simulink model "sys2"  (R2023b)
settings: Solver=VariableStepAuto  StartTime=0.0  StopTime=10.0  RelTol=1e-3
undefined symbols (not defined in the file): sys2
settings Model: Creator=lopez  LastModifiedBy=lopez

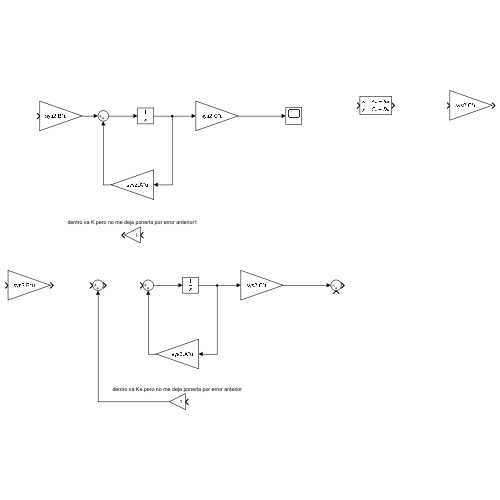
[thumbnail: Simulink's stored preview of the top-level diagram]
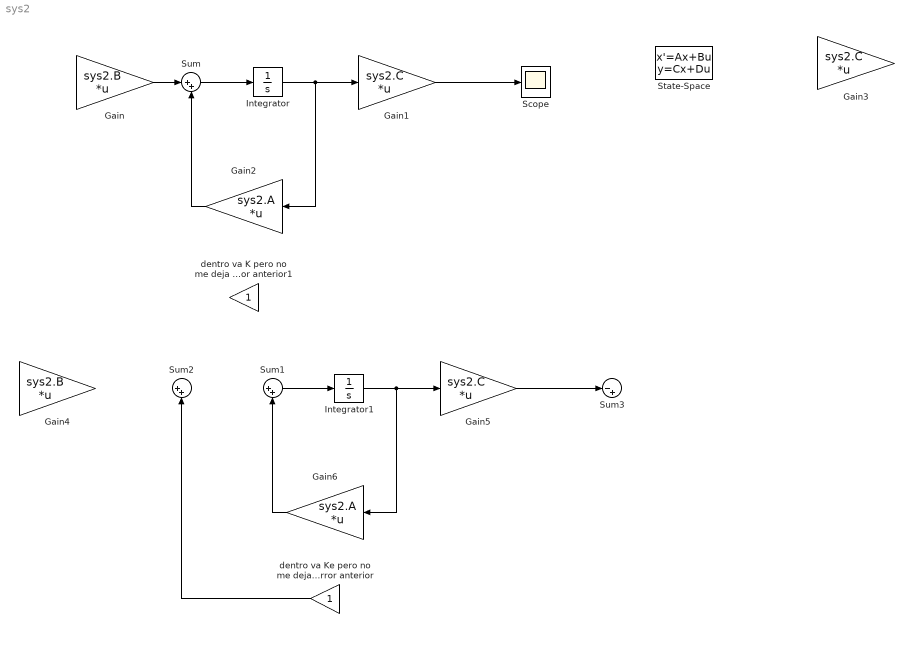
== system sys2 ==
  Gain : Gain  Gain=sys2.B  Multiplication=Matrix(K*u)
  Gain1 : Gain  Gain=sys2.C  Multiplication=Matrix(K*u)
  Gain2 : Gain  Gain=sys2.A  Multiplication=Matrix(K*u)
  Gain3 : Gain  Gain=sys2.C  Multiplication=Matrix(K*u)
  Gain4 : Gain  Gain=sys2.B  Multiplication=Matrix(K*u)
  Gain5 : Gain  Gain=sys2.C  Multiplication=Matrix(K*u)
  Gain6 : Gain  Gain=sys2.A  Multiplication=Matrix(K*u)
  Integrator : Integrator
  Integrator1 : Integrator
  Scope : Scope
  State-Space : StateSpace  A=sys2.A  B=sys2.B  C=sys2.C  D=sys2.D  InitialCondition=[1 0.1]
  Sum : Sum  Inputs=|++
  Sum1 : Sum  Inputs=|++
  Sum2 : Sum  Inputs=|++
  Sum3 : Sum  Inputs=|-+
  dentro va K pero no me deja ponerla por error anterior1 : Gain
  dentro va Ke pero no me deja ponerla por error anterior : Gain
  wires:
  Gain/1 -> Sum/1
  Sum/1 -> Integrator/1
  Integrator/1 -> Gain2/1, Gain1/1
  Gain2/1 -> Sum/2
  Gain1/1 -> Scope/1
  Sum1/1 -> Integrator1/1
  Gain6/1 -> Sum1/2
  Gain5/1 -> Sum3/1
  Integrator1/1 -> Gain6/1, Gain5/1
  dentro va Ke pero no me deja ponerla por error anterior/1 -> Sum2/2
